simulink model "VTOL_sim"  (R2016a)
settings: Solver=ode45  StartTime=0.0  StopTime=10000  RelTol=1e-3
InitFcn:
  | param
undefined symbols (not defined in the file or in its folder): drawVTOLsys
libraries: simulink x3
settings Model: Creator=beard  LastModifiedBy=Jacob
settings DataIOCC: LimitDataPoints=on  SaveFormat=Array  SignalLoggingSaveFormat=ModelDataLogs
settings OptimizationCC: ExpressionDepthLimit=2147483647  InitFltsAndDblsToZero=on
settings DebuggingCC: UnderspecifiedInitializationDetection=Classic  MergeDetectMultiDrivingBlocksExec=none  SolverPrmCheckMsg=warning  FcnCallInpInsideContextMsg=UseLocalSettings  StateNameClashWarn=warning
settings HardwareCC: ProdBitPerPointer=32  ProdLargestAtomicFloat=None  ProdIntDivRoundTo=Undefined  ProdEndianess=Unspecified  ProdWordSize=32  ProdHWDeviceType=32-bit Generic
settings ModelReferenceCC: PropagateSignalLabelsOutOfModel=off
settings GRTTargetCC: CombineOutputUpdateFcns=off  GRTInterface=on
settings ConfigComp: CovModelRefEnable=Off

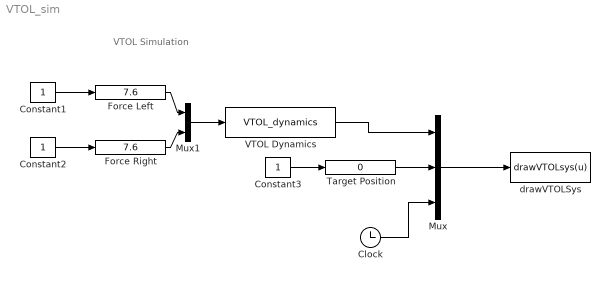
== system VTOL_sim ==
  note: VTOL Simulation
  Clock : Clock
  Constant1 : Constant
  Constant2 : Constant
  Constant3 : Constant
  Force Left : simulink/Math Operations/Slider Gain  low=7.35  gain=7.6  high=7.6
  Force Right : simulink/Math Operations/Slider Gain  low=7.35  gain=7.6  high=7.6
  Mux : Mux  Inputs=3
  Mux1 : Mux  Inputs=2
  "Target Position " : simulink/Math Operations/Slider Gain  low=0  gain=0  high=20
  VTOL Dynamics : S-Function  FunctionName=VTOL_dynamics  Parameters=P  SFunctionDeploymentMode=off  EnableBusSupport=off
  drawVTOLSys : MATLABFcn  MATLABFcn=drawVTOLsys(u)  OutputDimensions=0  SampleTime=0.1
  wires:
  Constant1/1 -> Force Left/1
  Mux/1 -> drawVTOLSys/1
  VTOL Dynamics/1 -> Mux/1
  Clock/1 -> Mux/3
  Constant2/1 -> Force Right/1
  "Target Position "/1 -> Mux/2
  Constant3/1 -> "Target Position "/1
  Mux1/1 -> VTOL Dynamics/1
  Force Left/1 -> Mux1/1
  Force Right/1 -> Mux1/2
